simulink model "NandiniG_23EEM1S02_foc_3mli_working_fine_Moscap"  (R2024b)
settings: Solver=ode1  StartTime=0.0  StopTime=1  FixedStep=0.000001  MaxStep=1e-4  RelTol=1e-3
InitFcn:
  | fs=2000;
model workspace (MAT data in the model file):
  Vref = 440
  cutoff_frequency = 500
  damping_factor = 0.707
  fn = 100
  fs = 2000
  ma = 1
libraries: simulink x24, spsMosfetLib x12, spsVoltageMeasurementLib x10, spsDiodeLib x6, powerlib_extras x6, spsSeriesRLCBranchLib x4, spsCurrentMeasurementLib x3, slpidlib x3, spsIGBTDiodeLib x2, spsDCVoltageSourceLib x1, spsGroundLib x1, spsPermanentMagnetSynchronousMachineLib x1
(part 1 of 2)
settings Model: VariantFading=off  Creator=Admin  LastModifiedBy=INNAGOL2
settings SolverCC: ZeroCrossAlgorithm=Adaptive
settings DebuggingCC: MaskedZcDiagnostic=none  IgnoredZcDiagnostic=none
settings RTWCC: GPUComputeCapability=3.5

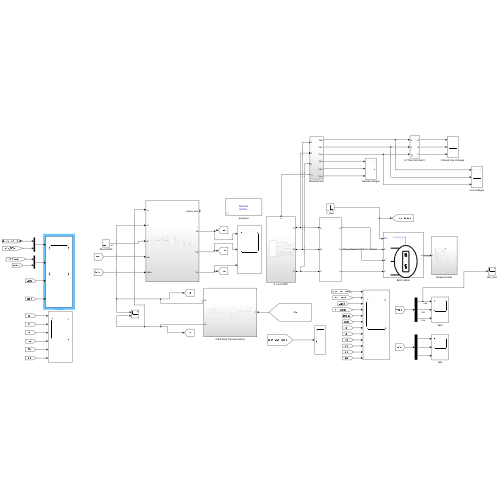
[thumbnail: Simulink's stored preview of the top-level diagram]
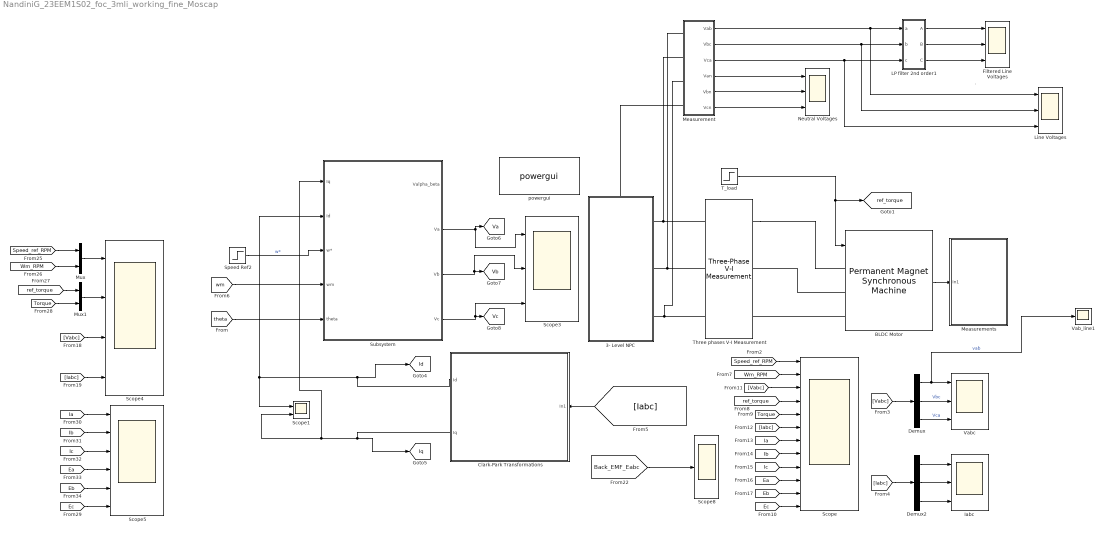
== system NandiniG_23EEM1S02_foc_3mli_working_fine_Moscap ==
  note: .
  3- Level NPC : Subsystem
      settings: PortSchema="{\"entries\":[{\"content\":{\"sides\":[{\"content\":{},\"type\":\"ConnectorPlacement.EquallySpacedRectSide\",\"uuid\":\"05cad51f-dea6-48e3-bce1-95addf868d22\"},{\"content\":{\"connectorIds\":[\"RConn1\",\"RConn2\",\"RConn3\"],\"side\":\"RIGHT\"},\"type\":\"ConnectorPlacement.EquallySpacedRectSide\",\"uuid\":\"1a16c647-6547-4e64-98e2-9e5b5587716a\"},{\"content\":{\"connectorIds\":[\"LConn1\"],\"side\":\"TOP\"},\"type\":\"ConnectorPlacement.EquallySpacedRectSide\",\"uuid\":\"a74f78e9-41fb-4fef-8e43-df7607ce5cf2\"}]},\"type\":\"ConnectorPlacement.EquallySpacedConnector\",\"uuid\":\"a99727e1-b578-4f76-a535-0af8e49f9bce\"}],\"packageUris\":[\"http://schema.mathworks.com/mf0/Connector/R2020b\"],\"version\":\"1.0\"}"
  BLDC Motor : spsPermanentMagnetSynchronousMachineLib/Permanent Magnet Synchronous Machine  NbPhases=3  FluxDistribution=Trapezoidal  RotorType=Round  MechanicalLoad=Torque Tm  PresetModel=No  ShowDetailedParameters=on  MeasurementBus=off  Resistance=0.7  Inductance=2.7e-3  dqInductances=[8.5e-3,8.5e-3]  La=0.000835  MachineConstant=Flux linkage established by magnets (V.s)  Flux=0.1194  VoltageCst=100.0283  TorqueCst=0.9552  Flat=120  Mechanical=[0.0027 0.0004924 4]  PolePairs=4  InitialConditions=[0,0, 0,0]  InitialConditions5ph=[0 0 0 0 0 0]  RefAngle=Aligned with phase A axis (original Park)  IterativeDiscreteModel=Trapezoidal non iterative  TsBlock=-1  TsPowergui=0
  Clark-Park Transformations : Subsystem
      settings: PortSchema="{\"entries\":[{\"content\":{\"sides\":[{\"content\":{\"connectorIds\":[\"Out1\",\"Out2\"]},\"type\":\"ConnectorPlacement.EquallySpacedRectSide\",\"uuid\":\"c290a13d-b4ce-440f-9d53-4b9274feb83f\"},{\"content\":{\"connectorIds\":[\"In1\"],\"side\":\"RIGHT\"},\"type\":\"ConnectorPlacement.EquallySpacedRectSide\",\"uuid\":\"3b8acf4d-0134-48df-ade6-fa9dd8548719\"},{\"content\":{\"side\":\"TOP\"},\"type\":\"ConnectorPlacement.EquallySpacedRectSide\",\"uuid\":\"08682ee2-bcb7-4f48-a64a-1997ed6d0a04\"}]},\"type\":\"ConnectorPlacement.EquallySpacedConnector\",\"uuid\":\"e640fd84-78ba-4bab-8695-1c4b1b64123a\"}],\"packageUris\":[\"http://schema.mathworks.com/mf0/Connector/R2020b\"],\"version\":\"1.0\"}"
  Demux : Demux  Outputs=3
  Demux2 : Demux  Outputs=3
  Filtered Line Voltages : Scope  NumInputPorts=3
  Iabc : Scope  NumInputPorts=3
  LP filter 2nd order1 : Subsystem  mask{cutoff_frequency=75, damping_factor=0.707}
      mask prompts: cutoff_frequency "Cut off frequency"; damping_factor "Damping Factor"
  Line Voltages : Scope  NumInputPorts=3
  Measurement : Subsystem
  Measurements : Subsystem
  Mux : Mux  Inputs=2
  Mux1 : Mux  Inputs=2
  Neutral Voltages : Scope  NumInputPorts=3
  Scope : Scope  NumInputPorts=12
  Scope1 : Scope  NumInputPorts=2
  Scope3 : Scope  NumInputPorts=3
  Scope4 : Scope  NumInputPorts=4
  Scope5 : Scope  NumInputPorts=6
  Scope8 : Scope
  Speed Ref2 : Step  Time=0.68  After=100  SampleTime=0
  Subsystem : Subsystem
  "T_load " : Step  Time=0.36  After=-5  SampleTime=0
  Three phases V-I Measurement : spsThreePhaseVIMeasurementLib/Three-Phase V-I Measurement  VoltageMeasurement=phase-to-phase  SetLabelV=on  LabelV=Vabc  Vpu=off  VpuLL=off  CurrentMeasurement=yes  SetLabelI=on  LabelI=Iabc  Ipu=off  Pbase=100e6  Vbase=500e3  OutputType=Complex  PhasorSimulation=off  PSBequivalent=0
  Vab_line1 : Scope
  Vabc : Scope  NumInputPorts=3
  powergui : spspowerguiLib/powergui  Priority=1  SimulationMode=Discrete  SampleTime=5e-05  frequency=60  Iterations=50  frequencyindice=0  Pbase=100e6  ErrMax=1e-4  UnitsV=kV  UnitsW=MW  buscounter=0  FunctionMessages=off  echomessages=off  EnableUseOfTLC=off  CurrentSourceSwitches=off  DisableSnubberDevices=off  DisableRonSwitches=off  DisableVfSwitches=off  DisplayEquations=off  AutomaticDiscreteSolvers=off  SolverType=Tustin/Backward Euler (TBE)  Interpol=off  ExternalGateDelay=off  methode=off  Ts=100  x0status=blocks  SPID=on  SwTol=0  HookPort=off  NonlinearTolerance=1e-4  nMaxIteration=100  ContinueOnMaxIteration=off  RestoreLinks=warning  ResistiveCurrentMeasurement=off  Frange=[0:2:500]  Ylog=off  Xlog=on  ShowGrid=off  save=off  variable=ZData  structure=0  ZoomFFT=off  StartTime=0.0  cycles=1  DisplayStyle=1  fundamental=60  FreqAxis=off  MaxFrequency=1000  frequencyindicesteady=1  RmsSteady=1  display=off
  tag scope: Id=global, Iq=global, Va=global, Vb=global, Vc=global, ref_torque=global
  wires:
  [Iabc] -> Clark-Park Transformations/1(In1)
  Clark-Park Transformations/1(Id) -> [Id], Scope1/1, Subsystem/2(Id)
  Clark-Park Transformations/2(Iq) -> Subsystem/1(Iq), Scope1/2, [Iq]
  [wm] -> Subsystem/4(wm)
  [theta] -> Subsystem/5(theta)
  Speed Ref2/1 -> Subsystem/3(w*)  "w*"
  "T_load "/1 -> BLDC Motor/1, [ref_torque]
  Subsystem/4(Vc) -> Scope3/3, [Vc]
  Subsystem/3(Vb) -> Scope3/2, [Vb]
  BLDC Motor/1 -> Measurements/1(In1)
  [Vabc] -> Scope/3
  [Ib] -> Scope/8
  [Ia] -> Scope/7
  [Ea] -> Scope/10
  [ref_torque] -> Scope/4
  [Ic] -> Scope/9
  [Ec] -> Scope/12
  [Eb] -> Scope/11
  [Torque] -> Scope/5
  [Wm_RPM] -> Scope/2
  [Iabc] -> Scope/6
  [Speed_ref_RPM] -> Scope/1
  Demux/3 -> Vabc/3  "Vca"
  Demux/2 -> Vabc/2  "Vbc"
  Demux/1 -> Vab_line1/1, Vabc/1  "vab"
  [Vabc] -> Demux/1
  [Iabc] -> Demux2/1
  Demux2/1 -> Iabc/1
  Demux2/3 -> Iabc/3
  Demux2/2 -> Iabc/2
  Subsystem/2(Va) -> [Va], Scope3/1
  [Iabc] -> Scope4/4
  [Vabc] -> Scope4/3
  Mux/1 -> Scope4/1
  [Speed_ref_RPM] -> Mux/1
  [Wm_RPM] -> Mux/2
  Mux1/1 -> Scope4/2
  [ref_torque] -> Mux1/1
  [Torque] -> Mux1/2
  [Ia] -> Scope5/1
  [Ib] -> Scope5/2
  [Ic] -> Scope5/3
  [Ea] -> Scope5/4
  [Eb] -> Scope5/5
  [Ec] -> Scope5/6
  [Back_EMF_Eabc] -> Scope8/1
  LP filter 2nd order1/3(C) -> Filtered Line Voltages/3
  LP filter 2nd order1/2(B) -> Filtered Line Voltages/2
  LP filter 2nd order1/1(A) -> Filtered Line Voltages/1
  Measurement/1(Vab) -> LP filter 2nd order1/1(a), Line Voltages/1
  Measurement/2(Vbc) -> Line Voltages/2, LP filter 2nd order1/2(b)
  Measurement/3(Vca) -> Line Voltages/3, LP filter 2nd order1/3(c)
  Measurement/4(Van) -> Neutral Voltages/1
  Measurement/5(Vbn) -> Neutral Voltages/2
  Measurement/6(Vcn) -> Neutral Voltages/3
  connections:
  BLDC Motor/LConn2 -- Three phases V-I Measurement/RConn2
  BLDC Motor/LConn3 -- Three phases V-I Measurement/RConn3
  Three phases V-I Measurement/RConn1 -- BLDC Motor/LConn1
  Three phases V-I Measurement/LConn3 -- Measurement/LConn3 -- 3- Level NPC/RConn3
  Three phases V-I Measurement/LConn2 -- Measurement/LConn1 -- 3- Level NPC/RConn2
  Three phases V-I Measurement/LConn1 -- Measurement/LConn2 -- 3- Level NPC/RConn1
  3- Level NPC/LConn1 -- Measurement/LConn4

== system NandiniG_23EEM1S02_foc_3mli_working_fine_Moscap/3- Level NPC ==
  NPC 3-level inverter : Subsystem
  " n" : PMIOPort  Side=Left
  A : PMIOPort  Port=2  Side=Right
  " B" : PMIOPort  Port=3  Side=Right
  " C" : PMIOPort  Port=4  Side=Right
  connections:
  NPC 3-level inverter/RConn2 -- " B"/RConn1
  NPC 3-level inverter/RConn1 -- A/RConn1
  NPC 3-level inverter/RConn3 -- " C"/RConn1
  " n"/RConn1 -- NPC 3-level inverter/RConn4

== system NandiniG_23EEM1S02_foc_3mli_working_fine_Moscap/Clark-Park Transformations ==
  In1 : Inport
  Demux1 : Demux  Outputs=3
  Scope3 : Scope  NumInputPorts=2
  Second-Order Filter1 : eeGeneralControl/Second-Order Filter  FilterType=Low-pass  fn=50  Zeta=0.707  Ts=-1  A0=0  Ph0=0  f0=0  b0=0
      settings: LibrarySourceBlock=ee_sl_lib/General Control/Second-Order Filter
  Subsystem : Subsystem
  Subsystem1 : Subsystem
  Id : Outport
  Iq : Outport  Port=2
  wires:
  Subsystem1/2(Iq) -> Iq/1, Scope3/2  "Iq"
  Subsystem1/1(Id) -> Id/1, Scope3/1  "Id"
  [theta] -> Subsystem1/3(theta)
  Subsystem/2(I_beta) -> Subsystem1/2(I_beta)
  Subsystem/1(I_alpha) -> Subsystem1/1(I_alpha)
  In1/1 -> Demux1/1
  Demux1/2 -> Subsystem/2(Ib)
  Demux1/1 -> Subsystem/1(Ia)
  Demux1/3 -> Subsystem/3(Ic)

== system NandiniG_23EEM1S02_foc_3mli_working_fine_Moscap/LP filter 2nd order1 ==
  a : Inport
  b : Inport  Port=2
  c : Inport  Port=3
  2nd-Order Filter : powerlib_extras/Control  Blocks/2nd-Order Filter  FilterType=Lowpass  Fo=cutoff_frequency  Zeta=damping_factor  Initialize=off  Vac_Init=[1 45 60]  Vdc_Init=-0.5  PlotResponse=off  param1=[1 500 1]
  2nd-Order Filter1 : powerlib_extras/Control  Blocks/2nd-Order Filter  FilterType=Lowpass  Fo=cutoff_frequency  Zeta=damping_factor  Initialize=off  Vac_Init=[1 45 60]  Vdc_Init=-0.5  PlotResponse=off  param1=[1 500 1]
  2nd-Order Filter2 : powerlib_extras/Control  Blocks/2nd-Order Filter  FilterType=Lowpass  Fo=cutoff_frequency  Zeta=damping_factor  Initialize=off  Vac_Init=[1 45 60]  Vdc_Init=-0.5  PlotResponse=off  param1=[1 500 1]
  A : Outport
  B : Outport  Port=2
  C : Outport  Port=3
  wires:
  2nd-Order Filter2/1 -> C/1
  c/1 -> 2nd-Order Filter2/1
  2nd-Order Filter1/1 -> B/1
  b/1 -> 2nd-Order Filter1/1
  2nd-Order Filter/1 -> A/1
  a/1 -> 2nd-Order Filter/1

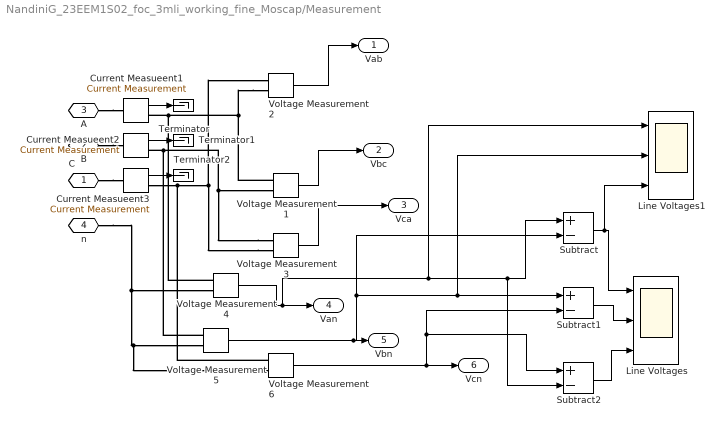
== system NandiniG_23EEM1S02_foc_3mli_working_fine_Moscap/Measurement ==
  Current Measueent1 : spsCurrentMeasurementLib/Current Measurement  PhasorSimulation=off  OutputType=Complex  PSBequivalent=0
  Current Measueent2 : spsCurrentMeasurementLib/Current Measurement  PhasorSimulation=off  OutputType=Complex  PSBequivalent=0
  Current Measueent3 : spsCurrentMeasurementLib/Current Measurement  PhasorSimulation=off  OutputType=Complex  PSBequivalent=0
  Line Voltages : Scope  NumInputPorts=3
  Line Voltages1 : Scope  NumInputPorts=3
  Subtract : Sum  Inputs=+-
  Subtract1 : Sum  Inputs=+-
  Subtract2 : Sum  Inputs=+-
  Terminator : Terminator
  Terminator1 : Terminator
  Terminator2 : Terminator
  Voltage Measurement{1..6} (6 alike) : spsVoltageMeasurementLib/Voltage Measurement  PhasorSimulation=off  OutputType=Complex  PSBequivalent=0
  C : PMIOPort  Side=Left
  B : PMIOPort  Port=2  Side=Left
  A : PMIOPort  Port=3  Side=Left
  " n" : PMIOPort  Port=4  Side=Left
  Vab : Outport
  Vbc : Outport  Port=2
  Vca : Outport  Port=3
  Van : Outport  Port=4
  Vbn : Outport  Port=5
  Vcn : Outport  Port=6
  wires:
  Current Measueent3/1 -> Terminator2/1
  Current Measueent2/1 -> Terminator1/1
  Current Measueent1/1 -> Terminator/1
  Voltage Measurement2/1 -> Vab/1
  Voltage Measurement1/1 -> Vbc/1
  Voltage Measurement3/1 -> Vca/1
  Voltage Measurement4/1 -> Line Voltages1/1, Subtract2/2, Subtract/1, Van/1
  Voltage Measurement5/1 -> Line Voltages1/2, Subtract1/1, Subtract/2, Vbn/1
  Voltage Measurement6/1 -> Subtract2/1, Subtract1/2, Vcn/1
  Subtract/1 -> Line Voltages1/3, Line Voltages/1
  Subtract1/1 -> Line Voltages/2
  Subtract2/1 -> Line Voltages/3
  connections:
  C/RConn1 -- Current Measueent3/LConn1
  B/RConn1 -- Current Measueent2/LConn1
  A/RConn1 -- Current Measueent1/LConn1
  Voltage Measurement3/LConn2 -- Voltage Measurement6/LConn1 -- Current Measueent3/RConn1 -- Voltage Measurement2/LConn1
  Voltage Measurement3/LConn1 -- Voltage Measurement5/LConn1 -- Current Measueent2/RConn1 -- Voltage Measurement1/LConn2
  Voltage Measurement2/LConn2 -- Voltage Measurement4/LConn1 -- Current Measueent1/RConn1 -- Voltage Measurement1/LConn1
  " n"/RConn1 -- Voltage Measurement6/LConn2 -- Voltage Measurement5/LConn2 -- Voltage Measurement4/LConn2

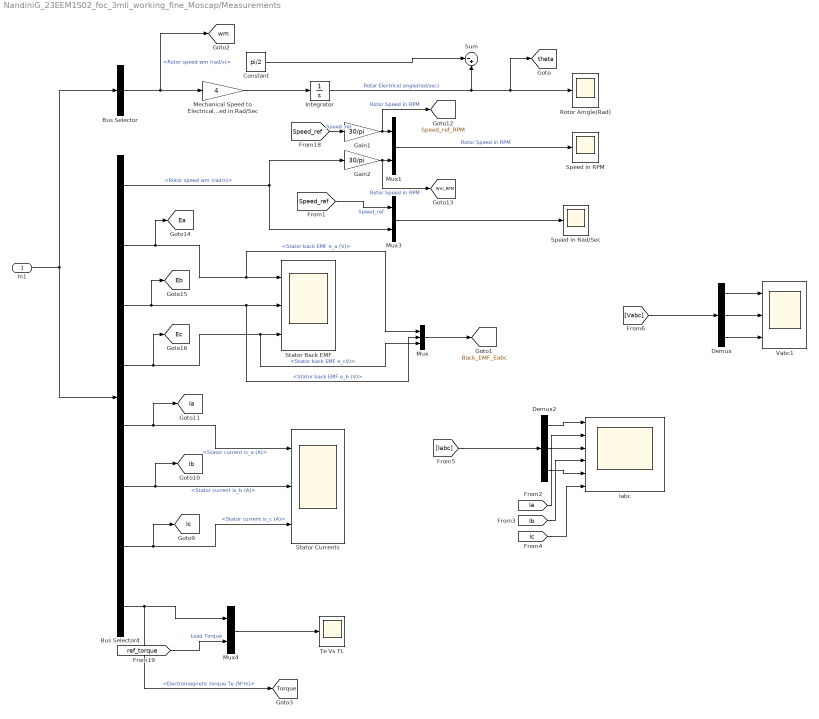
== system NandiniG_23EEM1S02_foc_3mli_working_fine_Moscap/Measurements ==
  In1 : Inport
  Bus Selector : BusSelector  OutputSignals=Rotor speed wm (rad/s)
  Bus Selector4 : BusSelector  OutputSignals=Rotor speed wm (rad/s),Stator back EMF e_a (V),Stator back EMF e_b (V),Stator back EMF e_cV),Stator current is_a (A),Stator current is_b (A),Stator current is_c (A),Electromagnetic torque Te (N*m)
  Constant : Constant  Value=pi/2
  Demux : Demux  Outputs=3
  Demux2 : Demux  Outputs=3
  Gain1 : Gain  Gain=30/pi
  Gain2 : Gain  Gain=30/pi
  Iabc : Scope  NumInputPorts=6
  Integrator : Integrator  WrapState=on
  Mechanical Speed to Electrical speed in Rad/Sec : Gain  Gain=4
  Mux : Mux  Inputs=3
  Mux1 : Mux  Inputs=2
  Mux3 : Mux  Inputs=2
  Mux4 : Mux  Inputs=2
  Rotor Amgle(Rad) : Scope
  Speed in RPM : Scope
  Speed in Rad/Sec : Scope
  Stator Back EMF : Scope  NumInputPorts=3
  Stator Currents : Scope  NumInputPorts=3
  Sum : Sum  Inputs=|-+
  Te Vs TL : Scope
  Vabc1 : Scope  NumInputPorts=3
  tag scope: Back_EMF_Eabc=global, Ea=global, Eb=global, Ec=global, Ia=global, Ib=global, Ic=global, Speed_ref_RPM=global, Torque=global, Wm_RPM=global, theta=global, wm=global
  wires:
  Bus Selector4/7 -> [Ic], Stator Currents/3  "<Stator current is_c (A)>"
  Bus Selector4/2 -> [Ea], Mux/1, Stator Back EMF/1  "<Stator back EMF e_a (V)>"
  Bus Selector/1 -> [wm], Mechanical Speed to Electrical speed in Rad/Sec/1  "<Rotor speed wm (rad/s)>"
  In1/1 -> Bus Selector4/1, Bus Selector/1
  Mux1/1 -> Speed in RPM/1  "Rotor Speed in RPM"
  Bus Selector4/5 -> [Ia], Stator Currents/1  "<Stator current is_a (A)>"
  [Speed_ref] -> Gain1/1  "Speed_ref"
  Gain2/1 -> [Wm_RPM], Mux1/2  "Rotor Speed in RPM"
  Bus Selector4/1 -> Mux3/2, Gain2/1  "<Rotor speed wm (rad/s)>"
  Mux3/1 -> Speed in Rad/Sec/1
  Bus Selector4/3 -> [Eb], Mux/2, Stator Back EMF/2  "<Stator back EMF e_b (V)>"
  Bus Selector4/8 -> [Torque], Mux4/1  "<Electromagnetic torque Te (N*m)>"
  Bus Selector4/4 -> [Ec], Mux/3, Stator Back EMF/3  "<Stator back EMF e_cV)>"
  [ref_torque] -> Mux4/2  "Load Torque"
  Bus Selector4/6 -> [Ib], Stator Currents/2  "<Stator current is_b (A)>"
  Mux4/1 -> Te Vs TL/1
  Mechanical Speed to Electrical speed in Rad/Sec/1 -> Integrator/1
  Gain1/1 -> [Speed_ref_RPM], Mux1/1  "Rotor Speed in RPM"
  [Speed_ref] -> Mux3/1  "Speed_ref"
  Integrator/1 -> [theta], Rotor Amgle(Rad)/1, Sum/2  "Rotar Electrical angle(rad/sec)"
  [Ib] -> Iabc/4
  [Ic] -> Iabc/6
  Demux2/2 -> Iabc/3
  Demux2/1 -> Iabc/1
  [Ia] -> Iabc/2
  Demux2/3 -> Iabc/5
  [Iabc] -> Demux2/1
  Mux/1 -> [Back_EMF_Eabc]
  Constant/1 -> Sum/1
  [Vabc] -> Demux/1
  Demux/1 -> Vabc1/1
  Demux/2 -> Vabc1/2
  Demux/3 -> Vabc1/3

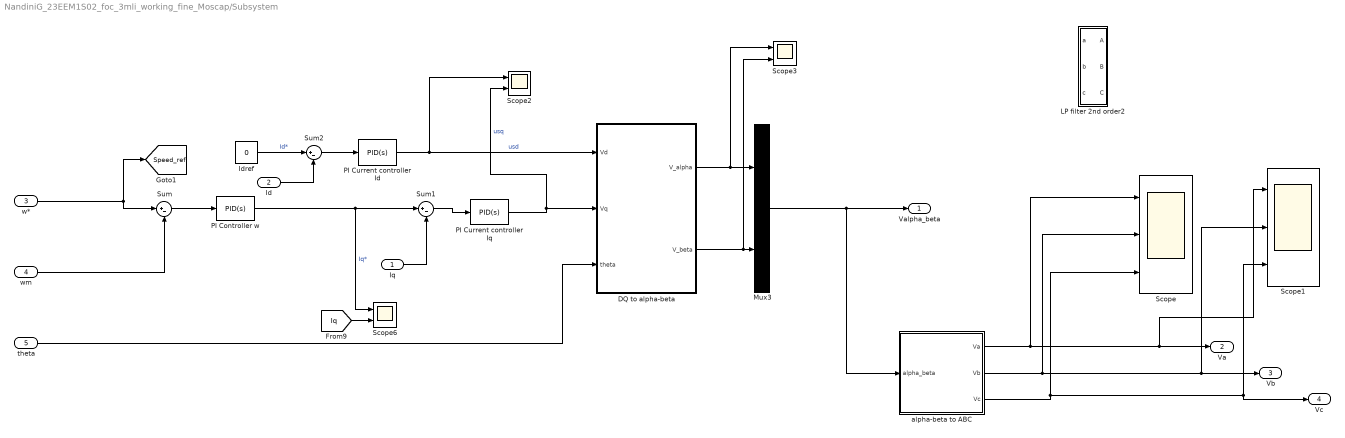
== system NandiniG_23EEM1S02_foc_3mli_working_fine_Moscap/Subsystem ==
  Iq : Inport
  Id : Inport  Port=2
  w* : Inport  Port=3
  wm : Inport  Port=4
  theta : Inport  Port=5
  DQ to alpha-beta : Subsystem
  Idref : Constant  Value=0
  LP filter 2nd order2 : Subsystem  mask{cutoff_frequency=500, damping_factor=0.707}
      mask prompts: cutoff_frequency "Cut off frequency"; damping_factor "Damping Factor"
  Mux3 : Mux  Inputs=2
  PI Controller w : slpidlib/PID Controller  Controller=PID  Form=Parallel  TimeDomain=Continuous-time  UseExternalTs=off  SampleTime=-1  IntegratorMethod=Forward Euler  FilterMethod=Forward Euler  ControllerParametersSource=internal  P=8  I=17  UseKiTs=off  D=0  UseExternalDerivativeSource=off  N=100  UseFilter=on  TunerSelectOption=Frequency Response Based  InitialConditionSource=internal  InitialConditionForIntegrator=0  InitialConditionForFilter=0  DifferentiatorICPrevScaledInput=0  ExternalReset=none  TrackingMode=off  Kt=1  LimitOutput=on  SatLimitsSource=internal  UpperSaturationLimit=80  LowerSaturationLimit=-80  LinearizeAsGain=on  AntiWindupMode=none  Kb=1  LimitIntegrator=on  UpperIntegratorSaturationLimit=80  LowerIntegratorSaturationLimit=-80  POutMin=[]  POutMax=[]  IOutMin=[]  IOutMax=[]  DOutMin=[]  DOutMax=[]  NOutMin=[]  NOutMax=[]  SumOutMin=[]  SumOutMax=[]  SaturationOutMin=[]  SaturationOutMax=[]  PParamMin=[]  PParamMax=[]  IParamMin=[]  IParamMax=[]  DParamMin=[]  DParamMax=[]  NParamMin=[]  NParamMax=[]  KbParamMin=[]  KbParamMax=[]  KtParamMin=[]  KtParamMax=[]  KbOutMin=[]  KbOutMax=[]  KtOutMin=[]  KtOutMax=[]  IntegratorOutMin=[]  IntegratorOutMax=[]  FilterOutMin=[]  FilterOutMax=[]  SumI1OutMin=[]  SumI1OutMax=[]  SumI2OutMin=[]  SumI2OutMax=[]  SumI3OutMin=[]  SumI3OutMax=[]  SumI4OutMin=[]  SumI4OutMax=[]  SumDOutMin=[]  SumDOutMax=[]  DifferentiatorOutMin=[]  DifferentiatorOutMax=[]  FilterDiffOutCoefMin=[]  FilterDiffOutCoefMax=[]  ReciprocalOutMin=[]  ReciprocalOutMax=[]  SumDenOutMin=[]  SumDenOutMax=[]  SumNumOutMin=[]  SumNumOutMax=[]  DivideOutMin=[]  DivideOutMax=[]  UdiffTsProdOutMin=[]  UdiffTsProdOutMax=[]  NTsProdOutMin=[]  NTsProdOutMax=[]  UintegralTsProdOutMin=[]  UintegralTsProdOutMax=[]  UngainTsProdOutMin=[]  UngainTsProdOutMax=[]  ClampingZeroOutDataTypeStr=Inherit: Inherit via back propagation  ClampingZeroOutMin=[]  ClampingZeroOutMax=[]  FilterDenConstantOutDataTypeStr=Inherit: Inherit via back propagation  FilterDenConstantOutMin=[]  FilterDenConstantOutMax=[]  PCopyOutDataTypeStr=Inherit: Inherit via back propagation  PCopyOutMin=[]  PCopyOutMax=[]  NCopyOutDataTypeStr=Inherit: Inherit via back propagation  NCopyOutMin=[]  NCopyOutMax=[]  IntegratorContinuousStateAttributes=''  IntegratorStateMustResolveToSignalObject=off  IntegratorRTWStateStorageClass=Auto  FilterContinuousStateAttributes=''  FilterStateMustResolveToSignalObject=off  FilterRTWStateStorageClass=Auto  ParallelPVariant=InternalParameters  IdealPVariant=Disabled  IVariant=InternalParameters  DVariant=InternalParameters  IntegratorVariant=Continuous  SatVariant=Enabled  AWVariant=Passthrough  PCopyVariant=Disabled  TRVariant=Disabled  FdbkBlocksVariant=Forward  IdealPFdbkVariant=Disabled  SatFdbkVariant=Disabled  DerivativeFilterVariant=ContFilter  NVariant=InternalParameters  NCopyVariant=Disabled  FilterICVariant=InternalICsFilter  IntegratorICVariant=InternalICs  ExternalResetVariant=Disabled  TRSumVariant=Passthrough  SumFdbkVariant=Disabled  SumVariant=Sum_PID  TsampFilterVariant=InternalTs  TsampNgainVariant=Passthrough  TsampIntegralVariant=Disabled_SignalSpec  ExternalSaturationOutDataTypeStr=Inherit: Same as second input  DerivativeSourceVariant=ErrorSignal  PreIntVariant=InternalPreInt
  PI Current controller Id : slpidlib/PID Controller  Controller=PID  Form=Parallel  TimeDomain=Continuous-time  UseExternalTs=off  SampleTime=-1  IntegratorMethod=Forward Euler  FilterMethod=Forward Euler  ControllerParametersSource=internal  P=2  I=1000  UseKiTs=off  D=0  UseExternalDerivativeSource=off  N=100  UseFilter=on  TunerSelectOption=Transfer Function Based (PID Tuner App)  InitialConditionSource=internal  InitialConditionForIntegrator=0  InitialConditionForFilter=0  DifferentiatorICPrevScaledInput=0  ExternalReset=none  TrackingMode=off  Kt=1  LimitOutput=on  SatLimitsSource=internal  UpperSaturationLimit=22  LowerSaturationLimit=-22  LinearizeAsGain=on  AntiWindupMode=clamping  Kb=1  LimitIntegrator=off  UpperIntegratorSaturationLimit=650  LowerIntegratorSaturationLimit=-650  POutMin=[]  POutMax=[]  IOutMin=[]  IOutMax=[]  DOutMin=[]  DOutMax=[]  NOutMin=[]  NOutMax=[]  SumOutMin=[]  SumOutMax=[]  SaturationOutMin=[]  SaturationOutMax=[]  PParamMin=[]  PParamMax=[]  IParamMin=[]  IParamMax=[]  DParamMin=[]  DParamMax=[]  NParamMin=[]  NParamMax=[]  KbParamMin=[]  KbParamMax=[]  KtParamMin=[]  KtParamMax=[]  KbOutMin=[]  KbOutMax=[]  KtOutMin=[]  KtOutMax=[]  IntegratorOutMin=[]  IntegratorOutMax=[]  FilterOutMin=[]  FilterOutMax=[]  SumI1OutMin=[]  SumI1OutMax=[]  SumI2OutMin=[]  SumI2OutMax=[]  SumI3OutMin=[]  SumI3OutMax=[]  SumI4OutMin=[]  SumI4OutMax=[]  SumDOutMin=[]  SumDOutMax=[]  DifferentiatorOutMin=[]  DifferentiatorOutMax=[]  FilterDiffOutCoefMin=[]  FilterDiffOutCoefMax=[]  ReciprocalOutMin=[]  ReciprocalOutMax=[]  SumDenOutMin=[]  SumDenOutMax=[]  SumNumOutMin=[]  SumNumOutMax=[]  DivideOutMin=[]  DivideOutMax=[]  UdiffTsProdOutMin=[]  UdiffTsProdOutMax=[]  NTsProdOutMin=[]  NTsProdOutMax=[]  UintegralTsProdOutMin=[]  UintegralTsProdOutMax=[]  UngainTsProdOutMin=[]  UngainTsProdOutMax=[]  ClampingZeroOutDataTypeStr=Inherit: Inherit via back propagation  ClampingZeroOutMin=[]  ClampingZeroOutMax=[]  FilterDenConstantOutDataTypeStr=Inherit: Inherit via back propagation  FilterDenConstantOutMin=[]  FilterDenConstantOutMax=[]  PCopyOutDataTypeStr=Inherit: Inherit via back propagation  PCopyOutMin=[]  PCopyOutMax=[]  NCopyOutDataTypeStr=Inherit: Inherit via back propagation  NCopyOutMin=[]  NCopyOutMax=[]  IntegratorContinuousStateAttributes=''  IntegratorStateMustResolveToSignalObject=off  IntegratorRTWStateStorageClass=Auto  FilterContinuousStateAttributes=''  FilterStateMustResolveToSignalObject=off  FilterRTWStateStorageClass=Auto  ParallelPVariant=InternalParameters  IdealPVariant=Disabled  IVariant=InternalParameters  DVariant=InternalParameters  IntegratorVariant=Continuous  SatVariant=Enabled  AWVariant=ContClampingParallel  PCopyVariant=Disabled  TRVariant=Disabled  FdbkBlocksVariant=Forward  IdealPFdbkVariant=Disabled  SatFdbkVariant=Disabled  DerivativeFilterVariant=ContFilter  NVariant=InternalParameters  NCopyVariant=Disabled  FilterICVariant=InternalICsFilter  IntegratorICVariant=InternalICs  ExternalResetVariant=Disabled  TRSumVariant=Passthrough  SumFdbkVariant=Disabled  SumVariant=Sum_PID  TsampFilterVariant=InternalTs  TsampNgainVariant=Passthrough  TsampIntegralVariant=Disabled_SignalSpec  ExternalSaturationOutDataTypeStr=Inherit: Same as second input  DerivativeSourceVariant=ErrorSignal  PreIntVariant=InternalPreInt
  PI Current controller Iq : slpidlib/PID Controller  Controller=PID  Form=Parallel  TimeDomain=Continuous-time  UseExternalTs=off  SampleTime=-1  IntegratorMethod=Forward Euler  FilterMethod=Forward Euler  ControllerParametersSource=internal  P=2  I=1000  UseKiTs=off  D=0  UseExternalDerivativeSource=off  N=100  UseFilter=on  TunerSelectOption=Transfer Function Based (PID Tuner App)  InitialConditionSource=internal  InitialConditionForIntegrator=0  InitialConditionForFilter=0  DifferentiatorICPrevScaledInput=0  ExternalReset=none  TrackingMode=off  Kt=1  LimitOutput=on  SatLimitsSource=internal  UpperSaturationLimit=165  LowerSaturationLimit=-165  LinearizeAsGain=on  AntiWindupMode=clamping  Kb=1  LimitIntegrator=off  UpperIntegratorSaturationLimit=650  LowerIntegratorSaturationLimit=-650  POutMin=[]  POutMax=[]  IOutMin=[]  IOutMax=[]  DOutMin=[]  DOutMax=[]  NOutMin=[]  NOutMax=[]  SumOutMin=[]  SumOutMax=[]  SaturationOutMin=[]  SaturationOutMax=[]  PParamMin=[]  PParamMax=[]  IParamMin=[]  IParamMax=[]  DParamMin=[]  DParamMax=[]  NParamMin=[]  NParamMax=[]  KbParamMin=[]  KbParamMax=[]  KtParamMin=[]  KtParamMax=[]  KbOutMin=[]  KbOutMax=[]  KtOutMin=[]  KtOutMax=[]  IntegratorOutMin=[]  IntegratorOutMax=[]  FilterOutMin=[]  FilterOutMax=[]  SumI1OutMin=[]  SumI1OutMax=[]  SumI2OutMin=[]  SumI2OutMax=[]  SumI3OutMin=[]  SumI3OutMax=[]  SumI4OutMin=[]  SumI4OutMax=[]  SumDOutMin=[]  SumDOutMax=[]  DifferentiatorOutMin=[]  DifferentiatorOutMax=[]  FilterDiffOutCoefMin=[]  FilterDiffOutCoefMax=[]  ReciprocalOutMin=[]  ReciprocalOutMax=[]  SumDenOutMin=[]  SumDenOutMax=[]  SumNumOutMin=[]  SumNumOutMax=[]  DivideOutMin=[]  DivideOutMax=[]  UdiffTsProdOutMin=[]  UdiffTsProdOutMax=[]  NTsProdOutMin=[]  NTsProdOutMax=[]  UintegralTsProdOutMin=[]  UintegralTsProdOutMax=[]  UngainTsProdOutMin=[]  UngainTsProdOutMax=[]  ClampingZeroOutDataTypeStr=Inherit: Inherit via back propagation  ClampingZeroOutMin=[]  ClampingZeroOutMax=[]  FilterDenConstantOutDataTypeStr=Inherit: Inherit via back propagation  FilterDenConstantOutMin=[]  FilterDenConstantOutMax=[]  PCopyOutDataTypeStr=Inherit: Inherit via back propagation  PCopyOutMin=[]  PCopyOutMax=[]  NCopyOutDataTypeStr=Inherit: Inherit via back propagation  NCopyOutMin=[]  NCopyOutMax=[]  IntegratorContinuousStateAttributes=''  IntegratorStateMustResolveToSignalObject=off  IntegratorRTWStateStorageClass=Auto  FilterContinuousStateAttributes=''  FilterStateMustResolveToSignalObject=off  FilterRTWStateStorageClass=Auto  ParallelPVariant=InternalParameters  IdealPVariant=Disabled  IVariant=InternalParameters  DVariant=InternalParameters  IntegratorVariant=Continuous  SatVariant=Enabled  AWVariant=ContClampingParallel  PCopyVariant=Disabled  TRVariant=Disabled  FdbkBlocksVariant=Forward  IdealPFdbkVariant=Disabled  SatFdbkVariant=Disabled  DerivativeFilterVariant=ContFilter  NVariant=InternalParameters  NCopyVariant=Disabled  FilterICVariant=InternalICsFilter  IntegratorICVariant=InternalICs  ExternalResetVariant=Disabled  TRSumVariant=Passthrough  SumFdbkVariant=Disabled  SumVariant=Sum_PID  TsampFilterVariant=InternalTs  TsampNgainVariant=Passthrough  TsampIntegralVariant=Disabled_SignalSpec  ExternalSaturationOutDataTypeStr=Inherit: Same as second input  DerivativeSourceVariant=ErrorSignal  PreIntVariant=InternalPreInt
  Scope : Scope  NumInputPorts=3
  Scope1 : Scope  NumInputPorts=3
  Scope2 : Scope  NumInputPorts=2
  Scope3 : Scope  NumInputPorts=2
  Scope6 : Scope  NumInputPorts=2
  Sum : Sum  Inputs=|+-
  Sum1 : Sum  Inputs=|+-
  Sum2 : Sum  Inputs=|+-
  alpha-beta to ABC : Subsystem
  Valpha_beta : Outport
  Va : Outport  Port=2
  Vb : Outport  Port=3
  Vc : Outport  Port=4
  tag scope: Speed_ref=global
  wires:
  PI Controller w/1 -> Scope6/1, Sum1/1  "Iq*"
  theta/1 -> DQ to alpha-beta/3(theta)
  Idref/1 -> Sum2/1  "Id*"
  Sum1/1 -> PI Current controller Iq/1
  Sum2/1 -> PI Current controller Id/1
  Sum/1 -> PI Controller w/1
  w*/1 -> [Speed_ref], Sum/1
  [Iq] -> Scope6/2
  DQ to alpha-beta/1(V_alpha) -> Scope3/1, Mux3/1
  DQ to alpha-beta/2(V_beta) -> Scope3/2, Mux3/2
  Mux3/1 -> alpha-beta to ABC/1(alpha_beta), Valpha_beta/1
  Iq/1 -> Sum1/2
  wm/1 -> Sum/2
  Id/1 -> Sum2/2
  PI Current controller Iq/1 -> Scope2/2, DQ to alpha-beta/2(Vq)  "usq"
  PI Current controller Id/1 -> Scope2/1, DQ to alpha-beta/1(Vd)  "usd"
  alpha-beta to ABC/1(Va) -> Scope1/1, Va/1, Scope/1
  alpha-beta to ABC/2(Vb) -> Scope1/2, Vb/1, Scope/2
  alpha-beta to ABC/3(Vc) -> Vc/1, Scope1/3, Scope/3

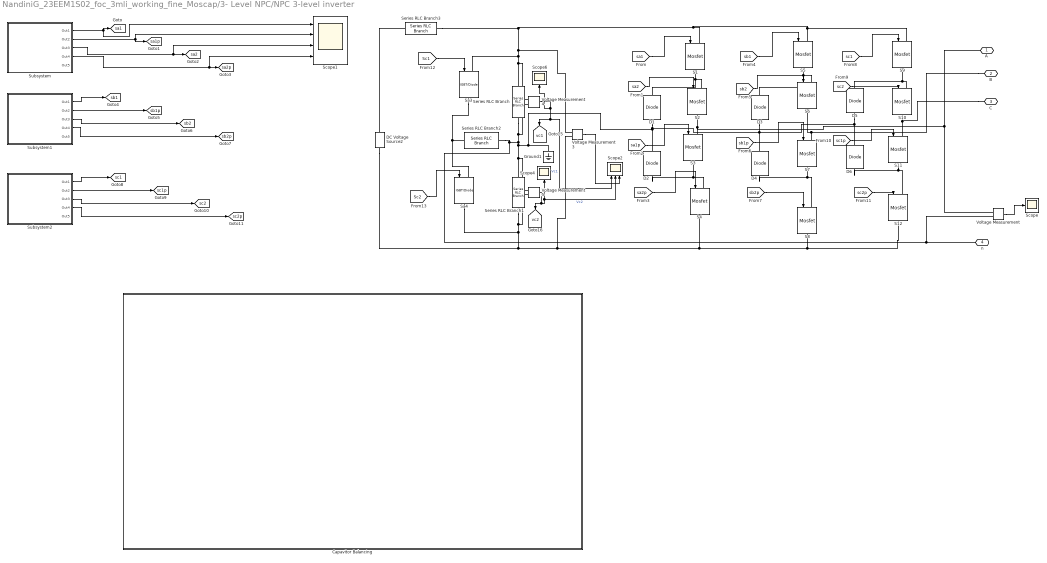
== system NandiniG_23EEM1S02_foc_3mli_working_fine_Moscap/3- Level NPC/NPC 3-level inverter ==
  Capavitor Balancing : Subsystem
  D{1..6} (6 alike) : spsDiodeLib/Diode  Ron=0.001  Lon=0  Vf=0.8  IC=0  UseSnubber=off  Rs=500  Cs=250e-9  Measurements=off
  DC Voltage Source2 : spsDCVoltageSourceLib/DC Voltage Source  Amplitude=160  Measurements=None
  Ground1 : spsGroundLib/Ground  LConnTagsString=a
  S{1..12} (12 alike) : spsMosfetLib/Mosfet  Ron=0.1  Lon=0  Rd=0.01  Vfd=0  IC=0  Rs=1e5  Cs=inf  Measurements=off
  Sa3 : spsIGBTDiodeLib/IGBT//Diode  Ron=1e-3  Rs=1e5  Cs=inf  Measurements=off
  Sa4 : spsIGBTDiodeLib/IGBT//Diode  Ron=1e-3  Rs=1e5  Cs=inf  Measurements=off
  Scope : Scope
  Scope1 : Scope  NumInputPorts=4
  Scope2 : Scope  NumInputPorts=3
  Scope4 : Scope
  Scope6 : Scope
  Series RLC Branch : spsSeriesRLCBranchLib/Series RLC Branch  LConnTagsString=__new0  RConnTagsString=__new0  BranchType=C  Resistance=1  Inductance=1e-3  SetiL0=off  InitialCurrent=0  Capacitance=4500e-6  Setx0=on  InitialVoltage=80  Measurements=None
  Series RLC Branch1 : spsSeriesRLCBranchLib/Series RLC Branch  LConnTagsString=__new0  RConnTagsString=__new0  BranchType=C  Resistance=1  Inductance=1e-3  SetiL0=off  InitialCurrent=0  Capacitance=4500e-6  Setx0=on  InitialVoltage=80  Measurements=None
  Series RLC Branch2 : spsSeriesRLCBranchLib/Series RLC Branch  LConnTagsString=__new0  RConnTagsString=__new0  BranchType=RL  Resistance=1  Inductance=1e-3  SetiL0=off  InitialCurrent=0  Capacitance=1e-6  Setx0=off  InitialVoltage=0  Measurements=None
  Series RLC Branch3 : spsSeriesRLCBranchLib/Series RLC Branch  LConnTagsString=__new0  RConnTagsString=__new0  BranchType=R  Resistance=0.001  Inductance=1e-3  SetiL0=off  InitialCurrent=0  Capacitance=1e-6  Setx0=off  InitialVoltage=0  Measurements=None
  Subsystem : Subsystem
  Subsystem1 : Subsystem
  Subsystem2 : Subsystem
  Voltage Measurement{,3..5} (4 alike) : spsVoltageMeasurementLib/Voltage Measurement  PhasorSimulation=off  OutputType=Complex  PSBequivalent=0
  A : PMIOPort  Side=Right
  " B" : PMIOPort  Port=2  Side=Right
  " C" : PMIOPort  Port=3  Side=Right
  " n" : PMIOPort  Port=4  Side=Right
  tag scope: sa1=global, sa1p=global, sa2=global, sa2p=global, sb1=global, sb1p=global, sb2=global, sb2p=global, sc1=global, sc1p=global, sc2=global, sc2p=global, vc1=global, vc2=global
  wires:
  [sa1] -> S1/1
  [sa2] -> S2/1
  [sa1p] -> S3/1
  [sa2p] -> S4/1
  [sb1] -> S5/1
  [sb2] -> S6/1
  [sb1p] -> S7/1
  [sb2p] -> S8/1
  [sc1] -> S9/1
  [sc2] -> S10/1
  [sc1p] -> S11/1
  [sc2p] -> S12/1
  Subsystem/1(Out1) -> [sa1], Scope1/1
  Subsystem/2(Out2) -> [sa1p], Scope1/2
  Subsystem/3(Out3) -> Scope1/3, [sa2]
  Subsystem/4(Out4) -> Scope1/4, [sa2p]
  Subsystem1/4(Out4) -> [sb2p]
  Subsystem1/3(Out3) -> [sb2]
  Subsystem1/2(Out2) -> [sb1p]
  Subsystem1/1(Out1) -> [sb1]
  Subsystem2/1(Out1) -> [sc1]
  Subsystem2/2(Out2) -> [sc1p]
  Subsystem2/3(Out3) -> [sc2]
  Subsystem2/4(Out4) -> [sc2p]
  ? -> ?
  Voltage Measurement/1 -> Scope/1
  Voltage Measurement5/1 -> [vc2], Scope4/1, Scope2/2  "Vc2"
  Voltage Measurement3/1 -> Scope2/3
  Voltage Measurement4/1 -> [vc1], Scope2/1, Scope6/1  "Vc1"
  [Sc1] -> Sa3/1
  [Sc2] -> Sa4/1
  connections:
  D1/RConn1 -- S2/LConn1 -- S1/RConn1
  D2/LConn1 -- S3/RConn1 -- S4/LConn1
  D3/RConn1 -- S6/LConn1 -- S5/RConn1
  D4/LConn1 -- S8/LConn1 -- S7/RConn1
  D5/RConn1 -- S10/LConn1 -- S9/RConn1
  D6/LConn1 -- S12/LConn1 -- S11/RConn1
  " C"/RConn1 -- S11/LConn1 -- S10/RConn1
  " B"/RConn1 -- S7/LConn1 -- S6/RConn1
  Voltage Measurement5/LConn1 -- Voltage Measurement/LConn2 -- " n"/RConn1 -- Series RLC Branch2/RConn1 -- Series RLC Branch/RConn1 -- Voltage Measurement4/LConn2 -- Ground1/LConn1 -- D6/RConn1 -- D5/LConn1 -- D4/RConn1 -- D3/LConn1 -- D1/LConn1 -- D2/RConn1 -- Series RLC Branch1/LConn1
  Voltage Measurement/LConn1 -- A/RConn1 -- S2/RConn1 -- S3/LConn1
  S1/LConn1 -- Series RLC Branch3/LConn1 -- Voltage Measurement3/LConn1 -- Sa3/LConn1 -- Series RLC Branch/LConn1 -- Voltage Measurement4/LConn1 -- S9/LConn1 -- S5/LConn1
  Sa4/RConn1 -- Series RLC Branch1/RConn1 -- Voltage Measurement5/LConn2 -- DC Voltage Source2/LConn1 -- S12/RConn1 -- S8/RConn1 -- S4/RConn1 -- Voltage Measurement3/LConn2
  Series RLC Branch3/RConn1 -- DC Voltage Source2/RConn1
  Sa3/RConn1 -- Series RLC Branch2/LConn1 -- Sa4/LConn1

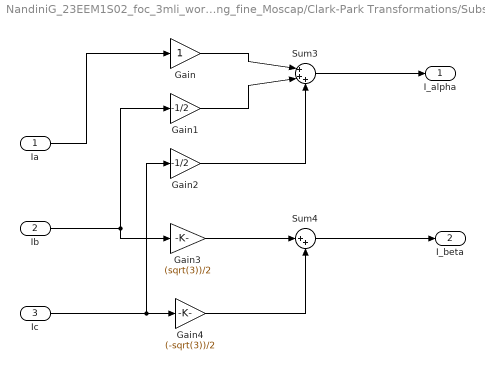
== system NandiniG_23EEM1S02_foc_3mli_working_fine_Moscap/Clark-Park Transformations/Subsystem ==
  Ia : Inport
  Ib : Inport  Port=2
  Ic : Inport  Port=3
  Gain : Gain
  Gain1 : Gain  Gain=-1/2
  Gain2 : Gain  Gain=-1/2
  Gain3 : Gain  Gain=(sqrt(3))/2
  Gain4 : Gain  Gain=(-sqrt(3))/2
  Sum3 : Sum  Inputs=|+++
  Sum4 : Sum  Inputs=|++
  I_alpha : Outport
  I_beta : Outport  Port=2
  wires:
  Gain2/1 -> Sum3/3
  Ib/1 -> Gain3/1, Gain1/1
  Sum3/1 -> I_alpha/1
  Gain3/1 -> Sum4/1
  Gain/1 -> Sum3/1
  Ic/1 -> Gain4/1, Gain2/1
  Gain1/1 -> Sum3/2
  Gain4/1 -> Sum4/2
  Ia/1 -> Gain/1
  Sum4/1 -> I_beta/1

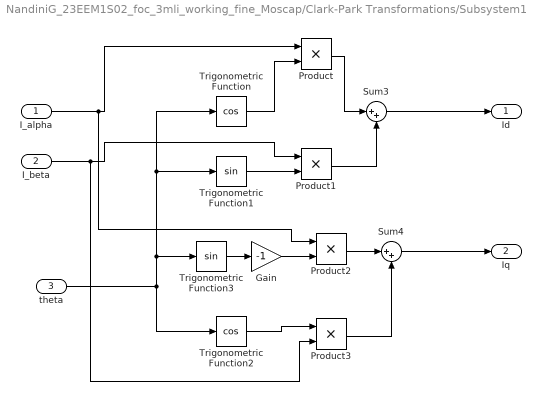
== system NandiniG_23EEM1S02_foc_3mli_working_fine_Moscap/Clark-Park Transformations/Subsystem1 ==
  I_alpha : Inport
  I_beta : Inport  Port=2
  theta : Inport  Port=3
  Gain : Gain  Gain=-1
  Product{,1..3} (4 alike) : Product
  Sum3 : Sum  Inputs=|++
  Sum4 : Sum  Inputs=|++
  Trigonometric Function : Trigonometry  Operator=cos
  Trigonometric Function1 : Trigonometry
  Trigonometric Function2 : Trigonometry  Operator=cos
  Trigonometric Function3 : Trigonometry
  Id : Outport
  Iq : Outport  Port=2
  wires:
  Sum3/1 -> Id/1
  Sum4/1 -> Iq/1
  Trigonometric Function3/1 -> Gain/1
  theta/1 -> Trigonometric Function2/1, Trigonometric Function3/1, Trigonometric Function1/1, Trigonometric Function/1
  Trigonometric Function/1 -> Product/2
  I_alpha/1 -> Product2/1, Product/1
  Trigonometric Function1/1 -> Product1/2
  I_beta/1 -> Product3/2, Product1/1
  Product/1 -> Sum3/1
  Product1/1 -> Sum3/2
  Gain/1 -> Product2/2
  Trigonometric Function2/1 -> Product3/1
  Product2/1 -> Sum4/1
  Product3/1 -> Sum4/2

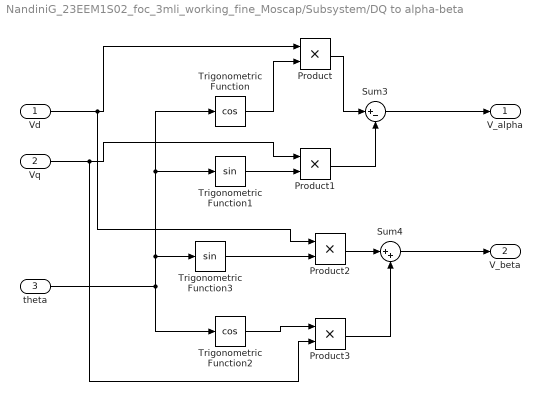
== system NandiniG_23EEM1S02_foc_3mli_working_fine_Moscap/Subsystem/DQ to alpha-beta ==
  Vd : Inport
  Vq : Inport  Port=2
  theta : Inport  Port=3
  Product{,1..3} (4 alike) : Product
  Sum3 : Sum  Inputs=|+-
  Sum4 : Sum  Inputs=|++
  Trigonometric Function : Trigonometry  Operator=cos
  Trigonometric Function1 : Trigonometry
  Trigonometric Function2 : Trigonometry  Operator=cos
  Trigonometric Function3 : Trigonometry
  V_alpha : Outport
  V_beta : Outport  Port=2
  wires:
  Product3/1 -> Sum4/2
  Product2/1 -> Sum4/1
  Trigonometric Function2/1 -> Product3/1
  Trigonometric Function3/1 -> Product2/2
  Product1/1 -> Sum3/2
  Product/1 -> Sum3/1
  Vq/1 -> Product1/1, Product3/2
  Trigonometric Function1/1 -> Product1/2
  Vd/1 -> Product/1, Product2/1
  Trigonometric Function/1 -> Product/2
  theta/1 -> Trigonometric Function/1, Trigonometric Function1/1, Trigonometric Function3/1, Trigonometric Function2/1
  Sum4/1 -> V_beta/1
  Sum3/1 -> V_alpha/1

== system NandiniG_23EEM1S02_foc_3mli_working_fine_Moscap/Subsystem/LP filter 2nd order2 ==
  a : Inport
  b : Inport  Port=2
  c : Inport  Port=3
  2nd-Order Filter : powerlib_extras/Control  Blocks/2nd-Order Filter  FilterType=Lowpass  Fo=cutoff_frequency  Zeta=damping_factor  Initialize=off  Vac_Init=[1 45 60]  Vdc_Init=-0.5  PlotResponse=off  param1=[1 500 1]
  2nd-Order Filter1 : powerlib_extras/Control  Blocks/2nd-Order Filter  FilterType=Lowpass  Fo=cutoff_frequency  Zeta=damping_factor  Initialize=off  Vac_Init=[1 45 60]  Vdc_Init=-0.5  PlotResponse=off  param1=[1 500 1]
  2nd-Order Filter2 : powerlib_extras/Control  Blocks/2nd-Order Filter  FilterType=Lowpass  Fo=cutoff_frequency  Zeta=damping_factor  Initialize=off  Vac_Init=[1 45 60]  Vdc_Init=-0.5  PlotResponse=off  param1=[1 500 1]
  A : Outport
  B : Outport  Port=2
  C : Outport  Port=3
  wires:
  a/1 -> 2nd-Order Filter/1
  2nd-Order Filter/1 -> A/1
  b/1 -> 2nd-Order Filter1/1
  2nd-Order Filter1/1 -> B/1
  c/1 -> 2nd-Order Filter2/1
  2nd-Order Filter2/1 -> C/1

== system NandiniG_23EEM1S02_foc_3mli_working_fine_Moscap/Subsystem/alpha-beta to ABC ==
  alpha_beta : Inport
  Demux : Demux  Outputs=2
  Gain5 : Gain  Gain=2/3
  Gain6 : Gain  Gain=1/sqrt(3)
  Gain7 : Gain  Gain=-1/3
  Gain8 : Gain  Gain=-1/3
  Gain9 : Gain  Gain=-1/sqrt(3)
  Sum1 : Sum  Inputs=|++
  Sum2 : Sum  Inputs=|++
  Va : Outport
  Vb : Outport  Port=2
  Vc : Outport  Port=3
  wires:
  Demux/1 -> Gain5/1, Gain8/1, Gain7/1
  Gain5/1 -> Va/1
  Demux/2 -> Gain9/1, Gain6/1
  Gain6/1 -> Sum1/1
  Gain7/1 -> Sum1/2
  Sum1/1 -> Vb/1
  Gain8/1 -> Sum2/1
  Gain9/1 -> Sum2/2
  Sum2/1 -> Vc/1
  alpha_beta/1 -> Demux/1

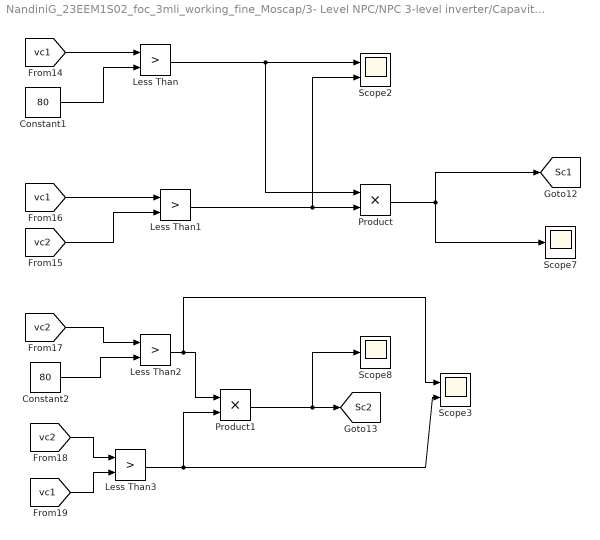
== system NandiniG_23EEM1S02_foc_3mli_working_fine_Moscap/3- Level NPC/NPC 3-level inverter/Capavitor Balancing ==
  Constant1 : Constant  Value=80
  Constant2 : Constant  Value=80
  Less Than{,1..3} (4 alike) : RelationalOperator  Operator=>  OutDataTypeStr=boolean  RndMeth=Simplest  InputSameDT=off
  Product : Product
  Product1 : Product
  Scope2 : Scope  NumInputPorts=2
  Scope3 : Scope  NumInputPorts=2
  Scope7 : Scope
  Scope8 : Scope
  tag scope: Sc1=global, Sc2=global
  wires:
  Product1/1 -> Scope8/1, [Sc2]
  Constant2/1 -> Less Than2/2
  Constant1/1 -> Less Than/2
  [vc1] -> Less Than3/2
  Product/1 -> Scope7/1, [Sc1]
  Less Than3/1 -> Scope3/2, Product1/2
  [vc2] -> Less Than1/2
  Less Than1/1 -> Scope2/2, Product/2
  [vc1] -> Less Than1/1
  Less Than2/1 -> Scope3/1, Product1/1
  Less Than/1 -> Product/1, Scope2/1
  [vc2] -> Less Than3/1
  [vc2] -> Less Than2/1
  [vc1] -> Less Than/1

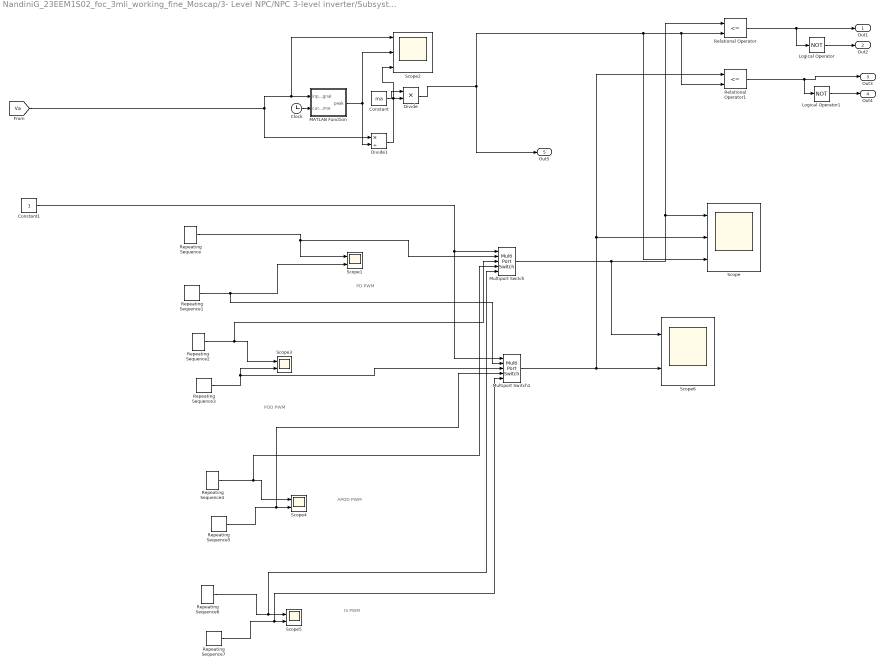
== system NandiniG_23EEM1S02_foc_3mli_working_fine_Moscap/3- Level NPC/NPC 3-level inverter/Subsystem ==
  note: IS PWM
  note: APOD PWM
  note: PD PWM
  note: POD PWM
  Clock : Clock
  Constant : Constant  Value=ma
  Constant1 : Constant
  Divide : Product  Inputs=**
  Divide1 : Product  Inputs=*/
  Logical Operator : Logic  Operator=NOT  AllPortsSameDT=off  OutDataTypeStr=boolean
  Logical Operator1 : Logic  Operator=NOT  AllPortsSameDT=off  OutDataTypeStr=boolean
  MATLAB Function : MATLAB Function  TreatAsAtomicUnit=on
  Multiport Switch : MultiPortSwitch  Inputs=4  SaturateOnIntegerOverflow=off  InputSameDT=off
  Multiport Switch1 : MultiPortSwitch  Inputs=4  SaturateOnIntegerOverflow=off  InputSameDT=off
  Relational Operator : RelationalOperator  Operator=<=  OutDataTypeStr=boolean  InputSameDT=off
  Relational Operator1 : RelationalOperator  Operator=<=  OutDataTypeStr=boolean  InputSameDT=off
  Repeating Sequence : simulink/Sources/Repeating Sequence  rep_seq_t=[0 0.25/fs 0.5/fs 0.75/fs 1/fs]  rep_seq_y=[0 0.5 1 0.5 0]
  Repeating Sequence1 : simulink/Sources/Repeating Sequence  rep_seq_t=[0 0.25/fs 0.5/fs 0.75/fs 1/fs]  rep_seq_y=[-1 -0.5 0 -0.5 -1]
  Repeating Sequence2 : simulink/Sources/Repeating Sequence  rep_seq_t=[0 0.25/fs 0.5/fs 0.75/fs 1/fs]  rep_seq_y=[0 0.5 1 0.5 0]
  Repeating Sequence3 : simulink/Sources/Repeating Sequence  rep_seq_t=[0 0.25/fs 0.5/fs 0.75/fs 1/fs]  rep_seq_y=[0 -0.5 -1 -0.5 0]
  Repeating Sequence4 : simulink/Sources/Repeating Sequence  rep_seq_t=[0 0.25/fs 0.5/fs 0.75/fs 1/fs]  rep_seq_y=[1 0.5 0 0.5 1]
  Repeating Sequence5 : simulink/Sources/Repeating Sequence  rep_seq_t=[0 0.25/fs 0.5/fs 0.75/fs 1/fs]  rep_seq_y=[-1 -0.5 0 -0.5 -1]
  Repeating Sequence6 : simulink/Sources/Repeating Sequence  rep_seq_t="[0  0.5/fs  1/fs]"  rep_seq_y="[-0.5  1  -0.5]"
  Repeating Sequence7 : simulink/Sources/Repeating Sequence  rep_seq_t="[0  0.5/fs  1/fs]"  rep_seq_y=[-1 0.5 -1]
  Scope : Scope  NumInputPorts=3
  Scope{1,3..6} (5 alike) : Scope  NumInputPorts=2
  Scope2 : Scope  NumInputPorts=3
  Out1 : Outport
  Out2 : Outport  Port=2
  Out3 : Outport  Port=3
  Out4 : Outport  Port=4
  Out5 : Outport  Port=5
  wires:
  Repeating Sequence1/1 -> Multiport Switch1/2, Scope1/2
  Repeating Sequence/1 -> Scope1/1, Multiport Switch/2
  Relational Operator1/1 -> Out3/1, Logical Operator1/1
  Relational Operator/1 -> Out1/1, Logical Operator/1
  Logical Operator1/1 -> Out4/1
  Logical Operator/1 -> Out2/1
  MATLAB Function/1(peak) -> Scope2/2, Divide1/2
  Clock/1 -> MATLAB Function/2(currentTime)
  Divide1/1 -> Scope2/3, Divide/2
  Constant/1 -> Divide/1
  Divide/1 -> Out5/1, Relational Operator/2, Relational Operator1/2, Scope/3
  [Va] -> Scope2/1, MATLAB Function/1(inputSignal), Divide1/1
  Repeating Sequence2/1 -> Multiport Switch/3, Scope3/1
  Repeating Sequence3/1 -> Multiport Switch1/3, Scope3/2
  Multiport Switch/1 -> Scope6/1, Relational Operator/1, Scope/1
  Multiport Switch1/1 -> Relational Operator1/1, Scope/2, Scope6/2
  Constant1/1 -> Multiport Switch1/1, Multiport Switch/1
  Repeating Sequence5/1 -> Multiport Switch1/4, Scope4/2
  Repeating Sequence4/1 -> Multiport Switch/4, Scope4/1
  Repeating Sequence7/1 -> Multiport Switch1/5, Scope5/2
  Repeating Sequence6/1 -> Multiport Switch/5, Scope5/1

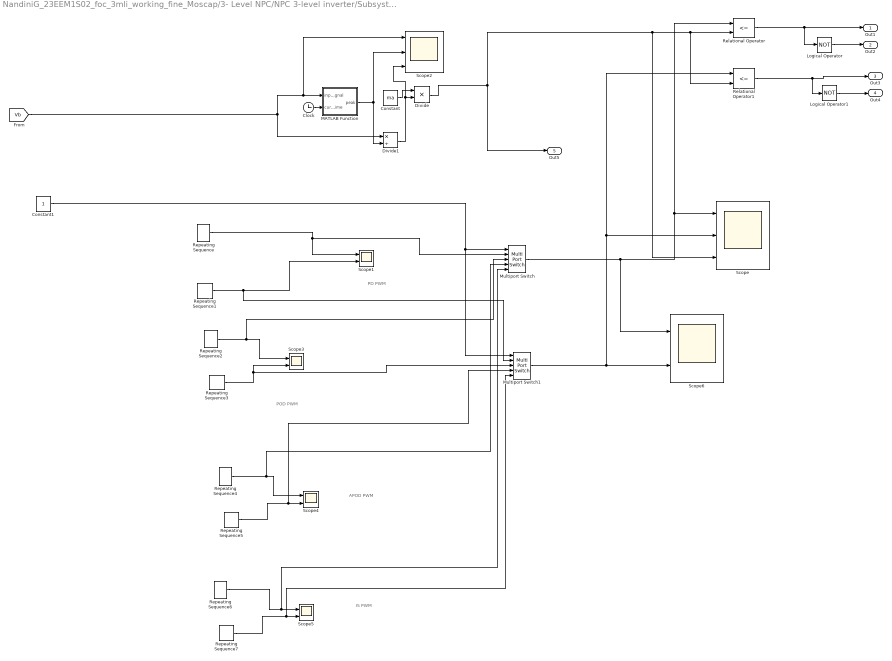
== system NandiniG_23EEM1S02_foc_3mli_working_fine_Moscap/3- Level NPC/NPC 3-level inverter/Subsystem1 ==
  note: IS PWM
  note: APOD PWM
  note: PD PWM
  note: POD PWM
  Clock : Clock
  Constant : Constant  Value=ma
  Constant1 : Constant
  Divide : Product  Inputs=**
  Divide1 : Product  Inputs=*/
  Logical Operator : Logic  Operator=NOT  AllPortsSameDT=off  OutDataTypeStr=boolean
  Logical Operator1 : Logic  Operator=NOT  AllPortsSameDT=off  OutDataTypeStr=boolean
  MATLAB Function : MATLAB Function  TreatAsAtomicUnit=on
  Multiport Switch : MultiPortSwitch  Inputs=4  SaturateOnIntegerOverflow=off  InputSameDT=off
  Multiport Switch1 : MultiPortSwitch  Inputs=4  SaturateOnIntegerOverflow=off  InputSameDT=off
  Relational Operator : RelationalOperator  Operator=<=  OutDataTypeStr=boolean  InputSameDT=off
  Relational Operator1 : RelationalOperator  Operator=<=  OutDataTypeStr=boolean  InputSameDT=off
  Repeating Sequence : simulink/Sources/Repeating Sequence  rep_seq_t=[0 0.25/fs 0.5/fs 0.75/fs 1/fs]  rep_seq_y=[0 0.5 1 0.5 0]
  Repeating Sequence1 : simulink/Sources/Repeating Sequence  rep_seq_t=[0 0.25/fs 0.5/fs 0.75/fs 1/fs]  rep_seq_y=[-1 -0.5 0 -0.5 -1]
  Repeating Sequence2 : simulink/Sources/Repeating Sequence  rep_seq_t=[0 0.25/fs 0.5/fs 0.75/fs 1/fs]  rep_seq_y=[0 0.5 1 0.5 0]
  Repeating Sequence3 : simulink/Sources/Repeating Sequence  rep_seq_t=[0 0.25/fs 0.5/fs 0.75/fs 1/fs]  rep_seq_y=[0 -0.5 -1 -0.5 0]
  Repeating Sequence4 : simulink/Sources/Repeating Sequence  rep_seq_t=[0 0.25/fs 0.5/fs 0.75/fs 1/fs]  rep_seq_y=[1 0.5 0 0.5 1]
  Repeating Sequence5 : simulink/Sources/Repeating Sequence  rep_seq_t=[0 0.25/fs 0.5/fs 0.75/fs 1/fs]  rep_seq_y=[-1 -0.5 0 -0.5 -1]
  Repeating Sequence6 : simulink/Sources/Repeating Sequence  rep_seq_t="[0  0.5/fs  1/fs]"  rep_seq_y="[-0.5  1  -0.5]"
  Repeating Sequence7 : simulink/Sources/Repeating Sequence  rep_seq_t="[0  0.5/fs  1/fs]"  rep_seq_y=[-1 0.5 -1]
  Scope : Scope  NumInputPorts=3
  Scope{1,3..6} (5 alike) : Scope  NumInputPorts=2
  Scope2 : Scope  NumInputPorts=3
  Out1 : Outport
  Out2 : Outport  Port=2
  Out3 : Outport  Port=3
  Out4 : Outport  Port=4
  Out5 : Outport  Port=5
  wires:
  Repeating Sequence6/1 -> Multiport Switch/5, Scope5/1
  Divide1/1 -> Scope2/3, Divide/2
  Repeating Sequence5/1 -> Multiport Switch1/4, Scope4/2
  MATLAB Function/1(peak) -> Scope2/2, Divide1/2
  Relational Operator1/1 -> Out3/1, Logical Operator1/1
  Clock/1 -> MATLAB Function/2(currentTime)
  [Vb] -> Scope2/1, MATLAB Function/1(inputSignal), Divide1/1
  Repeating Sequence1/1 -> Multiport Switch1/2, Scope1/2
  Repeating Sequence2/1 -> Multiport Switch/3, Scope3/1
  Multiport Switch/1 -> Scope6/1, Relational Operator/1, Scope/1
  Logical Operator1/1 -> Out4/1
  Repeating Sequence/1 -> Scope1/1, Multiport Switch/2
  Relational Operator/1 -> Out1/1, Logical Operator/1
  Repeating Sequence4/1 -> Multiport Switch/4, Scope4/1
  Constant1/1 -> Multiport Switch1/1, Multiport Switch/1
  Repeating Sequence7/1 -> Multiport Switch1/5, Scope5/2
  Divide/1 -> Out5/1, Relational Operator/2, Relational Operator1/2, Scope/3
  Multiport Switch1/1 -> Relational Operator1/1, Scope/2, Scope6/2
  Constant/1 -> Divide/1
  Repeating Sequence3/1 -> Multiport Switch1/3, Scope3/2
  Logical Operator/1 -> Out2/1

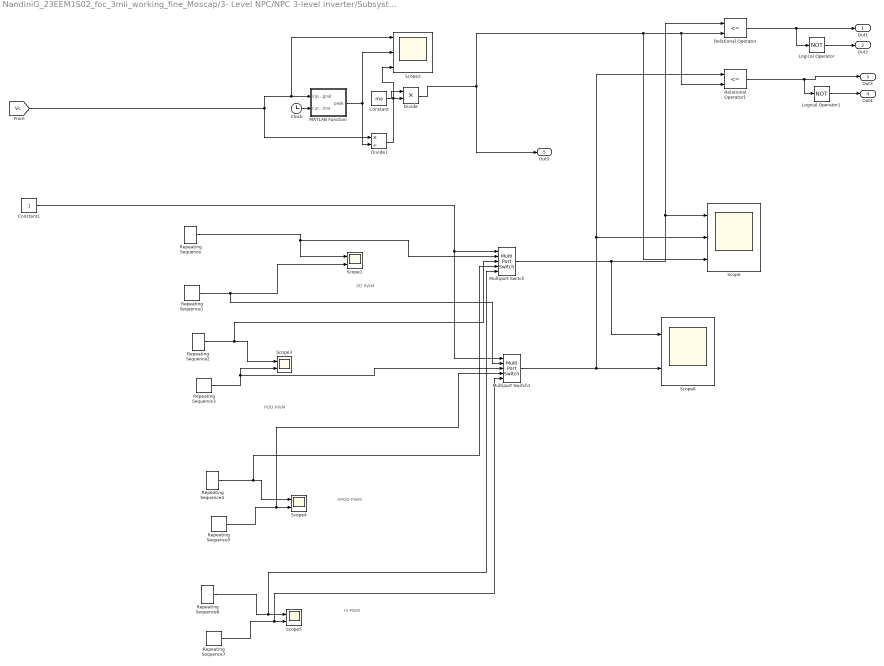
== system NandiniG_23EEM1S02_foc_3mli_working_fine_Moscap/3- Level NPC/NPC 3-level inverter/Subsystem2 ==
  note: IS PWM
  note: APOD PWM
  note: PD PWM
  note: POD PWM
  Clock : Clock
  Constant : Constant  Value=ma
  Constant1 : Constant
  Divide : Product  Inputs=**
  Divide1 : Product  Inputs=*/
  Logical Operator : Logic  Operator=NOT  AllPortsSameDT=off  OutDataTypeStr=boolean
  Logical Operator1 : Logic  Operator=NOT  AllPortsSameDT=off  OutDataTypeStr=boolean
  MATLAB Function : MATLAB Function  TreatAsAtomicUnit=on
  Multiport Switch : MultiPortSwitch  Inputs=4  SaturateOnIntegerOverflow=off  InputSameDT=off
  Multiport Switch1 : MultiPortSwitch  Inputs=4  SaturateOnIntegerOverflow=off  InputSameDT=off
  Relational Operator : RelationalOperator  Operator=<=  OutDataTypeStr=boolean  InputSameDT=off
  Relational Operator1 : RelationalOperator  Operator=<=  OutDataTypeStr=boolean  InputSameDT=off
  Repeating Sequence : simulink/Sources/Repeating Sequence  rep_seq_t=[0 0.25/fs 0.5/fs 0.75/fs 1/fs]  rep_seq_y=[0 0.5 1 0.5 0]
  Repeating Sequence1 : simulink/Sources/Repeating Sequence  rep_seq_t=[0 0.25/fs 0.5/fs 0.75/fs 1/fs]  rep_seq_y=[-1 -0.5 0 -0.5 -1]
  Repeating Sequence2 : simulink/Sources/Repeating Sequence  rep_seq_t=[0 0.25/fs 0.5/fs 0.75/fs 1/fs]  rep_seq_y=[0 0.5 1 0.5 0]
  Repeating Sequence3 : simulink/Sources/Repeating Sequence  rep_seq_t=[0 0.25/fs 0.5/fs 0.75/fs 1/fs]  rep_seq_y=[0 -0.5 -1 -0.5 0]
  Repeating Sequence4 : simulink/Sources/Repeating Sequence  rep_seq_t=[0 0.25/fs 0.5/fs 0.75/fs 1/fs]  rep_seq_y=[1 0.5 0 0.5 1]
  Repeating Sequence5 : simulink/Sources/Repeating Sequence  rep_seq_t=[0 0.25/fs 0.5/fs 0.75/fs 1/fs]  rep_seq_y=[-1 -0.5 0 -0.5 -1]
  Repeating Sequence6 : simulink/Sources/Repeating Sequence  rep_seq_t="[0  0.5/fs  1/fs]"  rep_seq_y="[-0.5  1  -0.5]"
  Repeating Sequence7 : simulink/Sources/Repeating Sequence  rep_seq_t="[0  0.5/fs  1/fs]"  rep_seq_y=[-1 0.5 -1]
  Scope : Scope  NumInputPorts=3
  Scope{1,3..6} (5 alike) : Scope  NumInputPorts=2
  Scope2 : Scope  NumInputPorts=3
  Out1 : Outport
  Out2 : Outport  Port=2
  Out3 : Outport  Port=3
  Out4 : Outport  Port=4
  Out5 : Outport  Port=5
  wires:
  Repeating Sequence6/1 -> Multiport Switch/5, Scope5/1
  Divide1/1 -> Scope2/3, Divide/2
  Repeating Sequence5/1 -> Multiport Switch1/4, Scope4/2
  MATLAB Function/1(peak) -> Scope2/2, Divide1/2
  Relational Operator1/1 -> Out3/1, Logical Operator1/1
  Clock/1 -> MATLAB Function/2(currentTime)
  [Vc] -> Scope2/1, MATLAB Function/1(inputSignal), Divide1/1
  Repeating Sequence1/1 -> Multiport Switch1/2, Scope1/2
  Repeating Sequence2/1 -> Multiport Switch/3, Scope3/1
  Multiport Switch/1 -> Scope6/1, Relational Operator/1, Scope/1
  Logical Operator1/1 -> Out4/1
  Repeating Sequence/1 -> Scope1/1, Multiport Switch/2
  Relational Operator/1 -> Out1/1, Logical Operator/1
  Repeating Sequence4/1 -> Multiport Switch/4, Scope4/1
  Constant1/1 -> Multiport Switch1/1, Multiport Switch/1
  Repeating Sequence7/1 -> Multiport Switch1/5, Scope5/2
  Divide/1 -> Out5/1, Relational Operator/2, Relational Operator1/2, Scope/3
  Multiport Switch1/1 -> Relational Operator1/1, Scope/2, Scope6/2
  Constant/1 -> Divide/1
  Repeating Sequence3/1 -> Multiport Switch1/3, Scope3/2
  Logical Operator/1 -> Out2/1

== matlab function NandiniG_23EEM1S02_foc_3mli_working_fine_Moscap/3- Level NPC/NPC 3-level inverter/Subsystem1/MATLAB Function ==
  settings: updateMethod=DISCRETE
  data: inputSignal input; peak output; currentTime input
function peak = getPeak(inputSignal, currentTime)
    % GETPEAK Function to track the peak value of a running waveform.
    %
    % INPUT:
    % inputSignal - Current sample of the waveform.
    % currentTime - Current simulation time.
    %
    % OUTPUT:
    % peak - The maximum absolute value encountered so far.
 
    % Persistent variables to store the peak values and the reset flag
    persistent maxPeak minPeak resetDone;
 
    % Initialize the persistent variables on the first function call
    if isempty(maxPeak)
        maxPeak = -inf;  % Start with a very low value
    end
    if isempty(minPeak)
        minPeak = inf;   % Start with a very high value
    end
    if isempty(resetDone)
        resetDone = false;  % Flag to indicate if reset has been done
    end
 
    % Reset the peak values once at 0.1 seconds
    if currentTime >= 0.11 && ~resetDone
        maxPeak = -inf;
        minPeak = inf;
        resetDone = true;  % Set the flag to true after reset
    end
 
    % Update the peak values if the current sample is larger or smaller
    if inputSignal > maxPeak
        maxPeak = inputSignal;
    end
    if inputSignal < minPeak
        minPeak = inputSignal;
    end
 
    % Calculate the peak-to-peak value
    peak = max(abs(maxPeak), abs(minPeak));
end

== matlab function NandiniG_23EEM1S02_foc_3mli_working_fine_Moscap/3- Level NPC/NPC 3-level inverter/Subsystem/MATLAB Function ==
  settings: updateMethod=DISCRETE
  data: inputSignal input; peak output; currentTime input
function peak = getPeak(inputSignal, currentTime)
    % GETPEAK Function to track the peak value of a running waveform.
    %
    % INPUT:
    % inputSignal - Current sample of the waveform.
    % currentTime - Current simulation time.
    %
    % OUTPUT:
    % peak - The maximum absolute value encountered so far.
 
    % Persistent variables to store the peak values and the reset flag
    persistent maxPeak minPeak resetDone;
 
    % Initialize the persistent variables on the first function call
    if isempty(maxPeak)
        maxPeak = -inf;  % Start with a very low value
    end
    if isempty(minPeak)
        minPeak = inf;   % Start with a very high value
    end
    if isempty(resetDone)
        resetDone = false;  % Flag to indicate if reset has been done
    end
 
    % Reset the peak values once at 0.1 seconds
    if currentTime >= 0.11 && ~resetDone
        maxPeak = -inf;
        minPeak = inf;
        resetDone = true;  % Set the flag to true after reset
    end
 
    % Update the peak values if the current sample is larger or smaller
    if inputSignal > maxPeak
        maxPeak = inputSignal;
    end
    if inputSignal < minPeak
        minPeak = inputSignal;
    end
 
    % Calculate the peak-to-peak value
    peak = max(abs(maxPeak), abs(minPeak));
end
